simulink model "Neurofeedback_Fuzzy_MISO_Full_cute"  (R2022a)
settings: Solver=VariableStepAuto  StartTime=0.0  StopTime=90  RelTol=1e-3
libraries: simulink x5, dspsrcs4 x4, fuzblock x1
settings Model: Creator=mdls3  LastModifiedBy=mariodelossantos

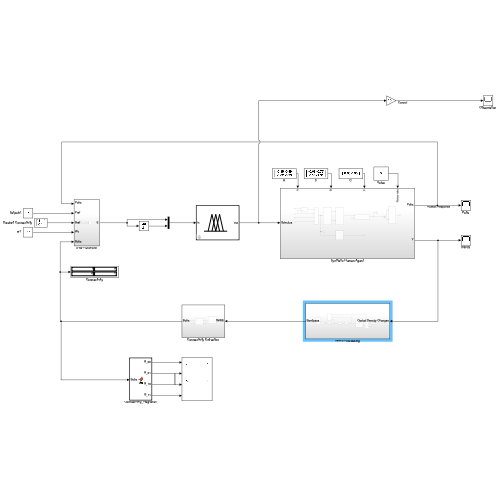
[thumbnail: Simulink's stored preview of the top-level diagram]
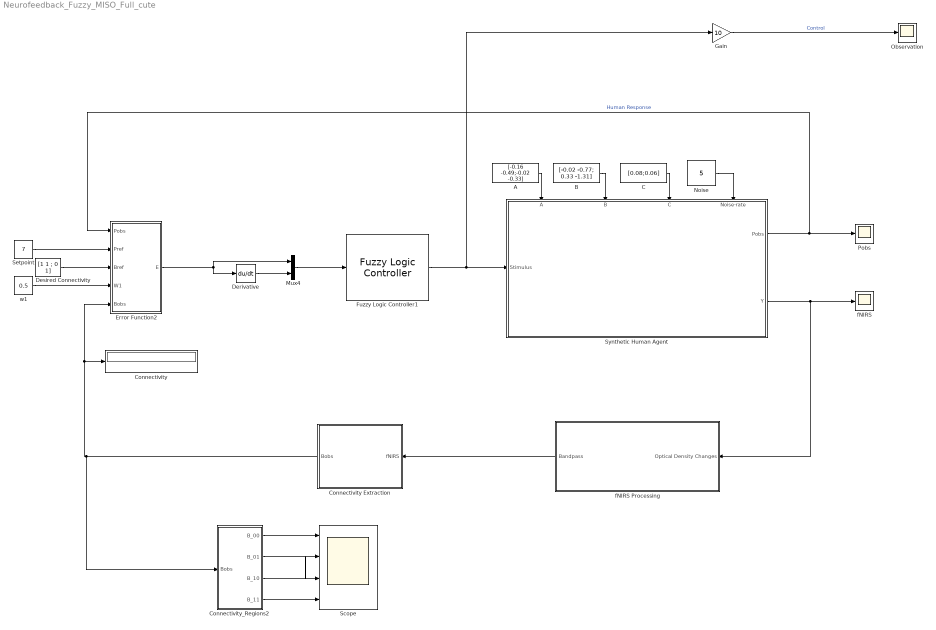
== system Neurofeedback_Fuzzy_MISO_Full_cute ==
  A : Constant  Value=[-0.16 -0.49;-0.02 -0.33]
  B : Constant  Value=[-0.02 -0.77; 0.33 -1.31]
  C : Constant  Value=[0.08;0.06]
  Connectivity : Display
  Connectivity Extraction : Subsystem
  Connectivity_Regions2 : MATLAB Function  TreatAsAtomicUnit=on
  Derivative : Derivative  CoefficientInTFapproximation=1
  Desired Connectivity : Constant  Value="[1   1 ; 0 1]"
  Error Function2 : Subsystem
  Fuzzy Logic Controller1 : fuzblock/Fuzzy Logic  Controller  FIS=cFNIRS_MISO_v3  OutputSampleNumber=101  DataType=double  FuzzifiedInputs=off  RuleFiringStrengths=off  RuleOutputs=off  AggregatedOutputs=off  SimulateUsing=Interpreted execution  OutOfRangeInputValueMessage=warning  NoRuleFiredMessage=warning  EmptyOutputFuzzySetMessage=warning
  Gain : Gain  Gain=10
  Mux4 : Mux  Inputs=2
  Noise : Constant  Value=5
  Observation : Scope
  Pobs : Scope
  Scope : Scope  NumInputPorts=4
  Setpoint : Constant  Value=7
  Synthetic Human Agent : Subsystem
      settings: PortSchema="{\"entries\":[{\"content\":{\"sides\":[{\"content\":{\"connectorIds\":[\"In1\"]},\"type\":\"ConnectorPlacement.EquallySpacedRectSide\",\"uuid\":\"bfbcc5e8-6241-430f-b542-d1842988c81e\"},{\"content\":{\"connectorIds\":[\"Out1\",\"Out2\"],\"side\":\"RIGHT\"},\"type\":\"ConnectorPlacement.EquallySpacedRectSide\",\"uuid\":\"5787ae13-1686-4c0f-bd71-92bd424cb6c3\"},{\"content\":{\"connectorIds\":[\"In2\",\"In3\",\"In4\",\"In5\"],\"side\":\"TOP\"},\"type\":\"ConnectorPlacement.EquallySpacedRectSide\",\"uuid\":\"d1dd531e-b262-408a-a912-471f5b03e825\"}]},\"type\":\"ConnectorPlacement.EquallySpacedConnector\",\"uuid\":\"b2c21004-90c2-4258-a219-9564d29dafe7\"}],\"packageUris\":[\"http://schema.mathworks.com/mf0/Connector/R2020b\"],\"version\":\"1.0\"}"
  fNIRS : Scope
  fNIRS Processing : Subsystem
  w1 : Constant  Value=0.5
  wires:
  Error Function2/1(E) -> Mux4/1, Derivative/1
  Synthetic Human Agent/2(Y) -> fNIRS/1, fNIRS Processing/1(Optical Density Changes)
  Noise/1 -> Synthetic Human Agent/5(Noise-rate)
  Derivative/1 -> Mux4/2
  Setpoint/1 -> Error Function2/2(Pref)
  Synthetic Human Agent/1(Pobs) -> Error Function2/1(Pobs), Pobs/1  "Human Response"
  Mux4/1 -> Fuzzy Logic Controller1/1
  A/1 -> Synthetic Human Agent/2(A)
  w1/1 -> Error Function2/4(W1)
  Desired Connectivity/1 -> Error Function2/3(Bref)
  C/1 -> Synthetic Human Agent/4(C)
  B/1 -> Synthetic Human Agent/3(B)
  Fuzzy Logic Controller1/1 -> Gain/1, Synthetic Human Agent/1(Stimulus)
  fNIRS Processing/1(Bandpass) -> Connectivity Extraction/1(fNIRS)
  Connectivity_Regions2/4(B_11) -> Scope/4
  Connectivity_Regions2/2(B_01) -> Scope/3
  Connectivity_Regions2/1(B_00) -> Scope/1
  Connectivity Extraction/1(Bobs) -> Connectivity_Regions2/1(Bobs), Error Function2/5(Bobs), Connectivity/1
  Connectivity_Regions2/3(B_10) -> Scope/2
  Gain/1 -> Observation/1  "Control"

== system Neurofeedback_Fuzzy_MISO_Full_cute/Connectivity Extraction ==
  fNIRS : Inport
  DQ1 : Scope
  Incremental_Avg_Boot1 : Subsystem
  Threshold : Constant  Value=0.6
  getConnectivity : MATLAB Function  TreatAsAtomicUnit=on  SystemSampleTime=0
  Bobs : Outport
  wires:
  getConnectivity/2(DQ) -> DQ1/1
  Incremental_Avg_Boot1/1("D ") -> getConnectivity/1("D ")
  Threshold/1 -> getConnectivity/2(Threshold)
  fNIRS/1 -> Incremental_Avg_Boot1/1(fNIRS)
  getConnectivity/1(Bobs) -> Bobs/1

== system Neurofeedback_Fuzzy_MISO_Full_cute/Error Function2 ==
  Pobs : Inport
  Pref : Inport  Port=2
  Bref : Inport  Port=3
  W1 : Inport  Port=4
  Bobs : Inport  Port=5
  Error Function : Subsystem
  Rehabilitation Train : Subsystem
  E : Outport
  wires:
  Bref/1 -> Error Function/3(Bref)
  Bobs/1 -> Error Function/4(Bobs)
  W1/1 -> Error Function/5(W1)
  Pref/1 -> Rehabilitation Train/1(In1)
  Pobs/1 -> Error Function/1(Pobs)
  Rehabilitation Train/1(Instruction) -> Error Function/2(Pref)
  Error Function/1(E) -> E/1

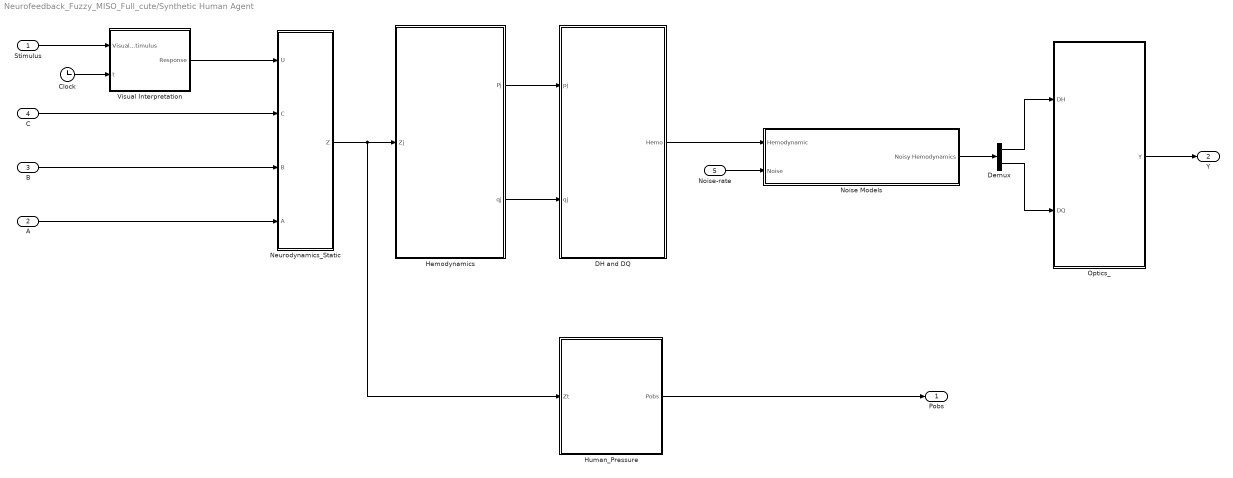
== system Neurofeedback_Fuzzy_MISO_Full_cute/Synthetic Human Agent ==
  Stimulus : Inport
  A : Inport  Port=2
  B : Inport  Port=3
  C : Inport  Port=4
  Noise-rate : Inport  Port=5
  Clock : Clock
  DH and DQ : Subsystem
  Demux : Demux  Outputs=2
  Hemodynamics : Subsystem
  Human_Pressure : Subsystem
  Neurodynamics_Static : Subsystem
  Noise Models : Subsystem
  Optics_ : MATLAB Function  TreatAsAtomicUnit=on
  Visual Interpretation : MATLAB Function  TreatAsAtomicUnit=on
  Pobs : Outport
  Y : Outport  Port=2
  wires:
  DH and DQ/1(Hemo) -> Noise Models/1(Hemodynamic)
  Hemodynamics/1(Pj) -> DH and DQ/1(pj)
  C/1 -> Neurodynamics_Static/2(C)
  Hemodynamics/2(qj) -> DH and DQ/2(qj)
  A/1 -> Neurodynamics_Static/4(A)
  Human_Pressure/1(Pobs) -> Pobs/1
  B/1 -> Neurodynamics_Static/3(B)
  Neurodynamics_Static/1(Z) -> Human_Pressure/1(Zt), Hemodynamics/1(Zj)
  Clock/1 -> Visual Interpretation/2(t)
  Stimulus/1 -> Visual Interpretation/1(Visual_Stimulus)
  Visual Interpretation/1(Response) -> Neurodynamics_Static/1(U)
  Noise Models/1(Noisy Hemodynamics) -> Demux/1
  Noise-rate/1 -> Noise Models/2(Noise)
  Demux/1 -> Optics_/1(DH)
  Demux/2 -> Optics_/2(DQ)
  Optics_/1(Y) -> Y/1

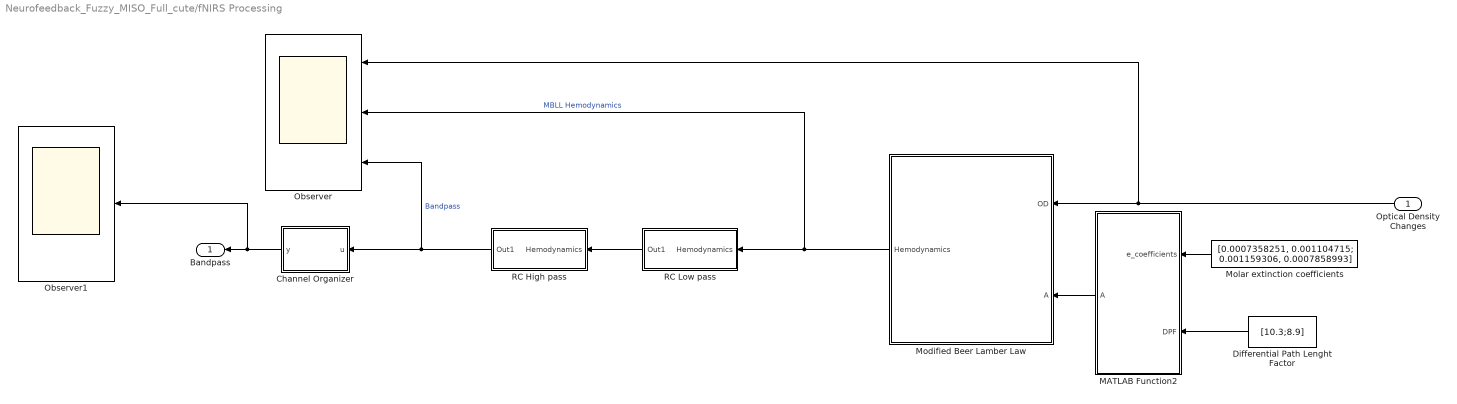
== system Neurofeedback_Fuzzy_MISO_Full_cute/fNIRS Processing ==
  Optical Density Changes : Inport
  Channel Organizer : MATLAB Function  TreatAsAtomicUnit=on
  Differential Path Lenght Factor : Constant  Value=[10.3;8.9]
  MATLAB Function2 : MATLAB Function  TreatAsAtomicUnit=on
  Modified Beer Lamber Law : MATLAB Function  TreatAsAtomicUnit=on
  Molar extinction coefficients : Constant  Value=|
      | [0.0007358251, 0.001104715;
      | 0.001159306, 0.0007858993]
  Observer : Scope  NumInputPorts=3
  Observer1 : Scope
  RC High pass : Subsystem
  RC Low pass : Subsystem
  Bandpass : Outport
  wires:
  Modified Beer Lamber Law/1(Hemodynamics) -> Observer/2, RC Low pass/1(Hemodynamics)  "MBLL Hemodynamics"
  Optical Density Changes/1 -> Modified Beer Lamber Law/1(OD), Observer/1
  RC High pass/1(Out1) -> Channel Organizer/1(u), Observer/3  "Bandpass"
  MATLAB Function2/1(A) -> Modified Beer Lamber Law/2(A)
  Differential Path Lenght Factor/1 -> MATLAB Function2/2(DPF)
  Molar extinction coefficients/1 -> MATLAB Function2/1(e_coefficients)
  Channel Organizer/1(y) -> Observer1/1, Bandpass/1
  RC Low pass/1(Out1) -> RC High pass/1(Hemodynamics)

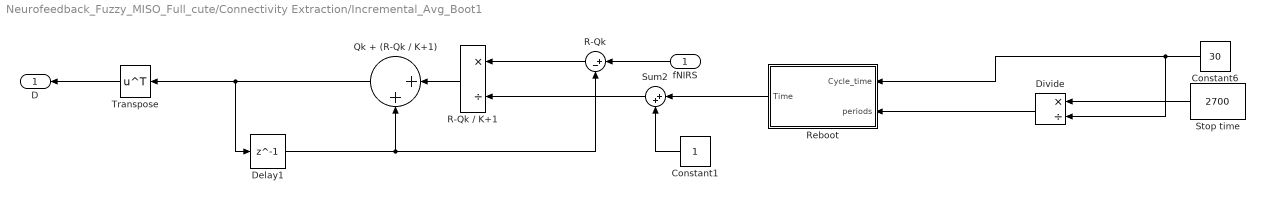
== system Neurofeedback_Fuzzy_MISO_Full_cute/Connectivity Extraction/Incremental_Avg_Boot1 ==
  fNIRS : Inport
  Constant1 : Constant
  Constant6 : Constant  Value=30
  Delay1 : Delay  DelayLength=1  InitialCondition=[0; 0; 0; 0]
  Divide : Product  Inputs=*/
  "Qk + (R-Qk / K+1) " : Sum  Inputs=|++
  R-Qk : Sum  Inputs=|+-
  R-Qk / K+1 : Product  Inputs=*/
  Reboot : Subsystem
  Stop time : Constant  Value=2700
  Sum2 : Sum  Inputs=|++
  Transpose : Math  Operator=transpose
  "D " : Outport
  wires:
  Constant1/1 -> Sum2/2
  fNIRS/1 -> R-Qk/1
  R-Qk / K+1/1 -> "Qk + (R-Qk / K+1) "/1
  Sum2/1 -> R-Qk / K+1/2
  R-Qk/1 -> R-Qk / K+1/1
  Delay1/1 -> R-Qk/2, "Qk + (R-Qk / K+1) "/2
  Reboot/1(Time) -> Sum2/1
  Constant6/1 -> Divide/2, Reboot/1(Cycle_time)
  Divide/1 -> Reboot/2(periods)
  Stop time/1 -> Divide/1
  "Qk + (R-Qk / K+1) "/1 -> Transpose/1, Delay1/1
  Transpose/1 -> "D "/1

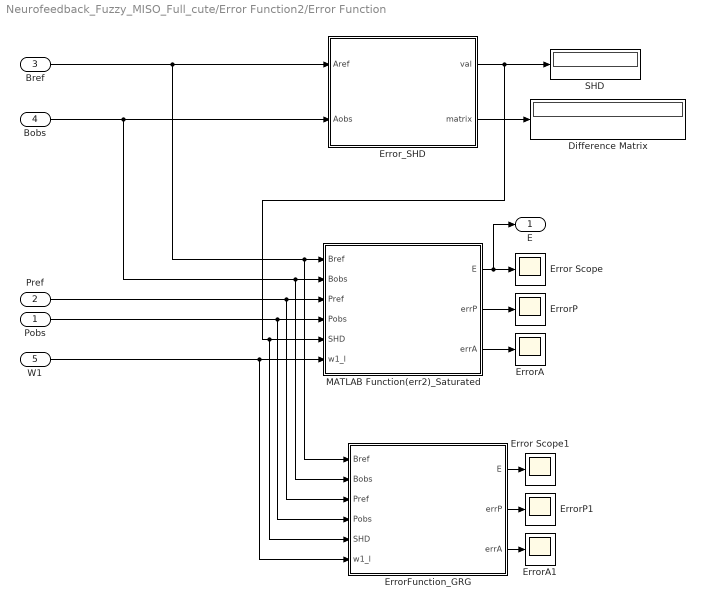
== system Neurofeedback_Fuzzy_MISO_Full_cute/Error Function2/Error Function ==
  Pobs : Inport
  Pref : Inport  Port=2
  Bref : Inport  Port=3
  Bobs : Inport  Port=4
  W1 : Inport  Port=5
  Difference Matrix : Display
  Error Scope : Scope
  Error Scope1 : Scope
  ErrorA : Scope
  ErrorA1 : Scope
  ErrorFunction_GRG : MATLAB Function  TreatAsAtomicUnit=on
  ErrorP : Scope
  ErrorP1 : Scope
  Error_SHD : MATLAB Function  TreatAsAtomicUnit=on
  MATLAB Function(err2)_Saturated : MATLAB Function  TreatAsAtomicUnit=on
  SHD : Display
  E : Outport
  wires:
  Error_SHD/2(matrix) -> Difference Matrix/1
  Bref/1 -> ErrorFunction_GRG/1(Bref), MATLAB Function(err2)_Saturated/1(Bref), Error_SHD/1(Aref)
  Error_SHD/1(val) -> ErrorFunction_GRG/5(SHD), MATLAB Function(err2)_Saturated/5(SHD), SHD/1
  Bobs/1 -> ErrorFunction_GRG/2(Bobs), MATLAB Function(err2)_Saturated/2(Bobs), Error_SHD/2(Aobs)
  Pref/1 -> ErrorFunction_GRG/3(Pref), MATLAB Function(err2)_Saturated/3(Pref)
  W1/1 -> MATLAB Function(err2)_Saturated/6(w1_l), ErrorFunction_GRG/6(w1_l)
  MATLAB Function(err2)_Saturated/1(E) -> E/1, Error Scope/1
  Pobs/1 -> ErrorFunction_GRG/4(Pobs), MATLAB Function(err2)_Saturated/4(Pobs)
  MATLAB Function(err2)_Saturated/2(errP) -> ErrorP/1
  MATLAB Function(err2)_Saturated/3(errA) -> ErrorA/1
  ErrorFunction_GRG/2(errP) -> ErrorP1/1
  ErrorFunction_GRG/3(errA) -> ErrorA1/1
  ErrorFunction_GRG/1(E) -> Error Scope1/1

== system Neurofeedback_Fuzzy_MISO_Full_cute/Error Function2/Rehabilitation Train ==
  In1 : Inport
  Duty_Cycle_U1 : Constant  Value=0.1666666666666667  OutMin=[0]  OutMax=[0.8]
  Period_Time_U1 : Constant  Value=30
  Setpoint_follow : Product
  Variable Pulse Generator2 : VariablePulseGenerator  AllowZeroPulseWidth=on  RunAtFixedTimeIntervals=on  SampleTime=1/10
  Instruction : Outport
  wires:
  Duty_Cycle_U1/1 -> Variable Pulse Generator2/1
  In1/1 -> Setpoint_follow/2
  Period_Time_U1/1 -> Variable Pulse Generator2/2
  Setpoint_follow/1 -> Instruction/1
  Variable Pulse Generator2/1 -> Setpoint_follow/1

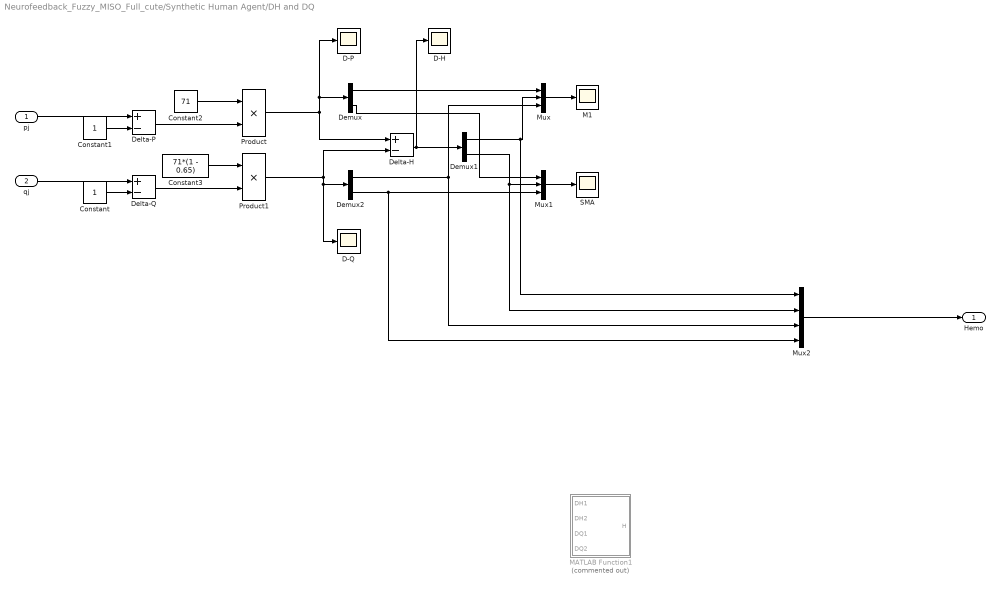
== system Neurofeedback_Fuzzy_MISO_Full_cute/Synthetic Human Agent/DH and DQ ==
  pj : Inport
  qj : Inport  Port=2
  Constant : Constant
  Constant1 : Constant
  Constant2 : Constant  Value=71
  Constant3 : Constant  Value=71*(1 - 0.65)
  D-H : Scope
  D-P : Scope
  D-Q : Scope
  Delta-H : Sum  Inputs=+-
  Delta-P : Sum  Inputs=+-
  Delta-Q : Sum  Inputs=+-
  Demux : Demux  Outputs=2
  Demux1 : Demux  Outputs=2
  Demux2 : Demux  Outputs=2
  M1 : Scope
  MATLAB Function1 : MATLAB Function  Commented=on  TreatAsAtomicUnit=on
  Mux : Mux  Inputs=3
  Mux1 : Mux  Inputs=3
  Mux2 : Mux
  Product : Product
  Product1 : Product
  SMA : Scope
  Hemo : Outport
  wires:
  Constant2/1 -> Product/1
  Delta-Q/1 -> Product1/2
  Constant3/1 -> Product1/1
  Demux2/2 -> Mux2/4, Mux1/3
  pj/1 -> Delta-P/1
  Mux1/1 -> SMA/1
  Demux/2 -> Mux1/1
  Mux/1 -> M1/1
  Constant/1 -> Delta-Q/2
  Delta-P/1 -> Product/2
  Product1/1 -> Demux2/1, D-Q/1, Delta-H/2
  qj/1 -> Delta-Q/1
  Demux/1 -> Mux/1
  Delta-H/1 -> Demux1/1, D-H/1
  Demux1/1 -> Mux2/1, Mux/2
  Demux1/2 -> Mux2/2, Mux1/2
  Product/1 -> Demux/1, D-P/1, Delta-H/1
  Demux2/1 -> Mux2/3, Mux/3
  Constant1/1 -> Delta-P/2
  Mux2/1 -> Hemo/1

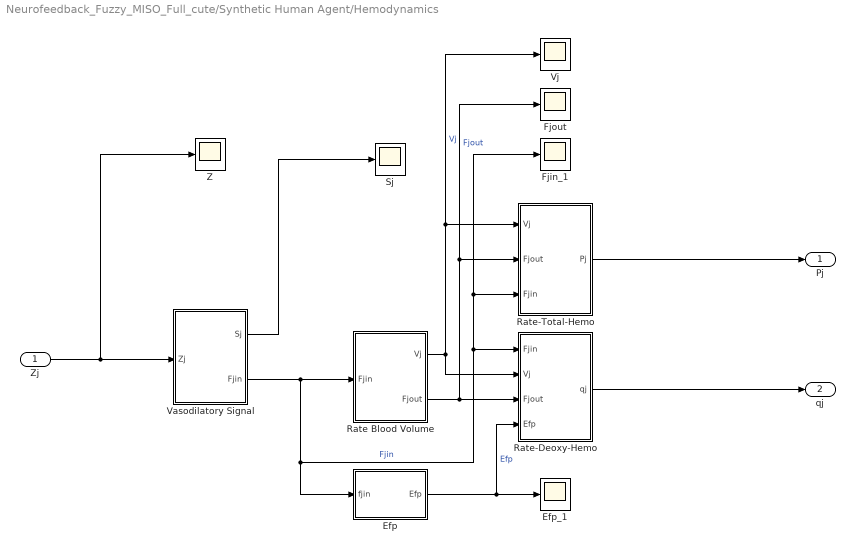
== system Neurofeedback_Fuzzy_MISO_Full_cute/Synthetic Human Agent/Hemodynamics ==
  Zj : Inport
  Efp : MATLAB Function  TreatAsAtomicUnit=on
  Efp_1 : Scope
  Fjin_1 : Scope
  Fjout : Scope
  Rate Blood Volume : Subsystem
  Rate-Deoxy-Hemo : Subsystem
  Rate-Total-Hemo : Subsystem
  Sj : Scope
  Vasodilatory Signal : Subsystem
  Vj : Scope
  Z : Scope
  Pj : Outport
  qj : Outport  Port=2
  wires:
  Rate-Deoxy-Hemo/1(qj) -> qj/1
  Zj/1 -> Vasodilatory Signal/1(Zj), Z/1
  Vasodilatory Signal/1(Sj) -> Sj/1
  Rate Blood Volume/2(Fjout) -> Fjout/1, Rate-Total-Hemo/2(Fjout), Rate-Deoxy-Hemo/3(Fjout)  "Fjout"
  Rate Blood Volume/1(Vj) -> Vj/1, Rate-Total-Hemo/1(Vj), Rate-Deoxy-Hemo/2(Vj)  "Vj"
  Rate-Total-Hemo/1(Pj) -> Pj/1
  Efp/1(Efp) -> Rate-Deoxy-Hemo/4(Efp), Efp_1/1  "Efp"
  Vasodilatory Signal/2(Fjin) -> Efp/1(fjin), Fjin_1/1, Rate-Total-Hemo/3(Fjin), Rate-Deoxy-Hemo/1(Fjin), Rate Blood Volume/1(Fjin)  "Fjin"

== system Neurofeedback_Fuzzy_MISO_Full_cute/Synthetic Human Agent/Human_Pressure ==
  Zt : Inport
  Clock : Clock
  Gain : Gain  Gain=10
  Pressure Generator : MATLAB Function  TreatAsAtomicUnit=on
  SENSOR : MATLAB Function  TreatAsAtomicUnit=on
  Scope : Scope
  Scope1 : Scope
  Pobs : Outport
  wires:
  Clock/1 -> Pressure Generator/2(t)
  Zt/1 -> Pressure Generator/1(Zt)
  SENSOR/1(Pobs) -> Scope1/1, Gain/1
  Pressure Generator/1(Pobs) -> SENSOR/1(Vout), Scope/1
  Gain/1 -> Pobs/1

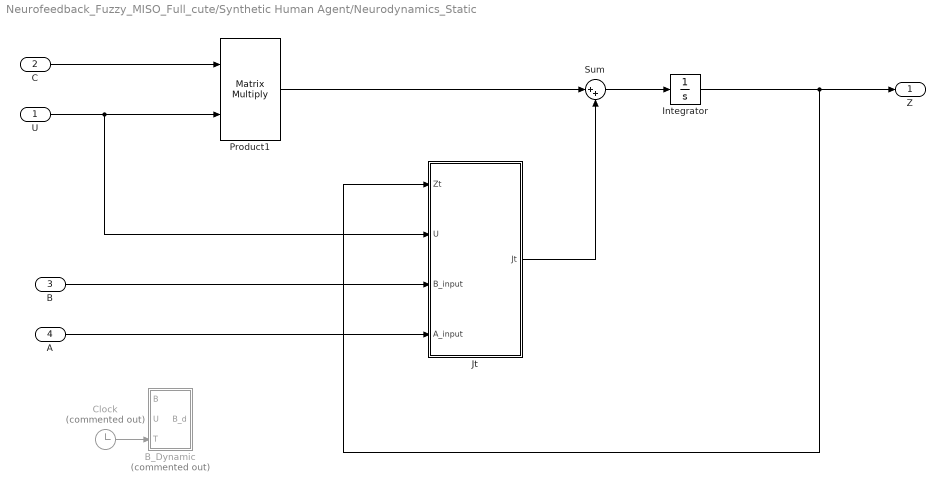
== system Neurofeedback_Fuzzy_MISO_Full_cute/Synthetic Human Agent/Neurodynamics_Static ==
  U : Inport
  C : Inport  Port=2
  B : Inport  Port=3
  A : Inport  Port=4
  B_Dynamic : Subsystem  Commented=on
  Clock : Clock  Commented=on
  Integrator : Integrator
  Jt : MATLAB Function  TreatAsAtomicUnit=on
  Product1 : Product  Multiplication=Matrix(*)
  Sum : Sum  Inputs=|++
  Z : Outport
  wires:
  Integrator/1 -> Jt/1(Zt), Z/1
  Product1/1 -> Sum/1
  Jt/1(Jt) -> Sum/2
  Sum/1 -> Integrator/1
  U/1 -> Product1/2, Jt/2(U)
  C/1 -> Product1/1
  A/1 -> Jt/4(A_input)
  Clock/1 -> B_Dynamic/3(T)
  B/1 -> Jt/3(B_input)

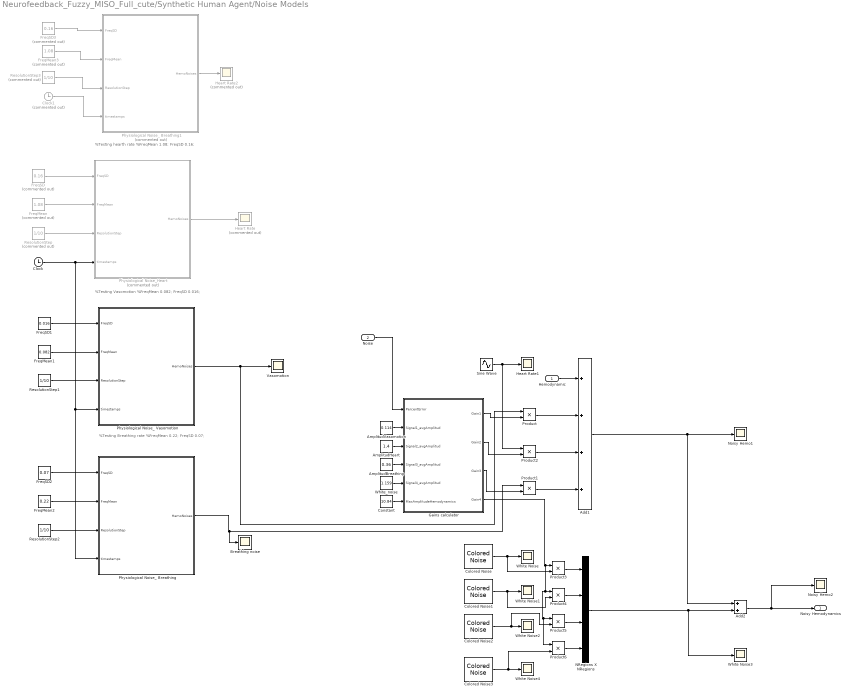
== system Neurofeedback_Fuzzy_MISO_Full_cute/Synthetic Human Agent/Noise Models ==
  note: %Testing hearth rate
      | %FreqMean 1.08; FreqSD 0.16;
  note: %Testing Breathing rate
      | %FreqMean 0.22; FreqSD 0.07;
  note: %Testing Vasomotion
      | %FreqMean 0.082; FreqSD 0.016;
  Hemodynamic : Inport
  Noise : Inport  Port=2
  Add1 : Sum  Inputs=++++
  Add2 : Sum
  AmplitudBreathing : Constant  Value=0.36
  AmplitudHeart : Constant  Value=1.4
  AmplitudVasomotion : Constant  Value=0.114
  Breathing noise : Scope
  Clock : Clock
  Clock1 : Clock  Commented=on
  Colored Noise : dspsrcs4/Colored Noise  Color=white  InverseFrequencyPower=1  BoundedOutput=on  NumChannels=1  OutputDataType=double  SamplesPerFrame=1  SampleTime=1/10  RandomStream=mt19937ar with seed  Seed=67  SimulateUsing=Interpreted execution
      settings: SourceProductBaseCode=DS
  Colored Noise1 : dspsrcs4/Colored Noise  Color=white  InverseFrequencyPower=1  BoundedOutput=on  NumChannels=1  OutputDataType=double  SamplesPerFrame=1  SampleTime=1/10  RandomStream=mt19937ar with seed  Seed=40  SimulateUsing=Interpreted execution
      settings: SourceProductBaseCode=DS
  Colored Noise2 : dspsrcs4/Colored Noise  Color=white  InverseFrequencyPower=1  BoundedOutput=on  NumChannels=1  OutputDataType=double  SamplesPerFrame=1  SampleTime=1/10  RandomStream=mt19937ar with seed  Seed=41  SimulateUsing=Interpreted execution
      settings: SourceProductBaseCode=DS
  Colored Noise3 : dspsrcs4/Colored Noise  Color=white  InverseFrequencyPower=1  BoundedOutput=on  NumChannels=1  OutputDataType=double  SamplesPerFrame=1  SampleTime=1/10  RandomStream=mt19937ar with seed  Seed=50  SimulateUsing=Interpreted execution
      settings: SourceProductBaseCode=DS
  Constant : Constant  Value=10.84
  FreqMean : Constant  Commented=on  Value=1.08
  FreqMean1 : Constant  Value=0.082
  FreqMean2 : Constant  Value=0.22
  FreqMean3 : Constant  Commented=on  Value=1.08
  FreqSD : Constant  Commented=on  Value=0.16
  FreqSD1 : Constant  Value=0.016
  FreqSD2 : Constant  Value=0.07
  FreqSD3 : Constant  Commented=on  Value=0.16
  Gains calculator : MATLAB Function  TreatAsAtomicUnit=on
  Heart Rate : Scope  Commented=on
  Heart Rate1 : Scope
  Heart Rate2 : Scope  Commented=on
  NRegions X NRegions : Mux
  Noisy Hemo1 : Scope
  Noisy Hemo2 : Scope
  Physiological Noise_ Breathing : MATLAB Function  TreatAsAtomicUnit=on
  Physiological Noise_ Breathing1 : MATLAB Function  Commented=on  TreatAsAtomicUnit=on
  Physiological Noise_ Vasomotion : MATLAB Function  TreatAsAtomicUnit=on
  Physiological Noise_Heart : MATLAB Function  Commented=on  TreatAsAtomicUnit=on
  Product{,1..6} (7 alike) : Product
  ResolutionStep : Constant  Commented=on  Value=1/10
  ResolutionStep1 : Constant  Value=1/10
  ResolutionStep2 : Constant  Value=1/10
  ResolutionStep3 : Constant  Commented=on  Value=1/10
  Sine Wave : Sin  Frequency=1.08 * 2*pi  SampleTime=0
  Vasomotion : Scope
  White Noise{,1..4} (5 alike) : Scope
  White_noise : Constant  Value=1.159
  Noisy Hemodynamics : Outport
  wires:
  FreqSD/1 -> Physiological Noise_Heart/1(FreqSD)
  FreqMean/1 -> Physiological Noise_Heart/2(FreqMean)
  ResolutionStep/1 -> Physiological Noise_Heart/3(ResolutionStep)
  ResolutionStep1/1 -> Physiological Noise_ Vasomotion/3(ResolutionStep)
  FreqSD1/1 -> Physiological Noise_ Vasomotion/1(FreqSD)
  Clock/1 -> Physiological Noise_Heart/4(timestamps), Physiological Noise_ Breathing/4(timestamps), Physiological Noise_ Vasomotion/4(timestamps)
  FreqMean1/1 -> Physiological Noise_ Vasomotion/2(FreqMean)
  Physiological Noise_ Breathing/1(HemoNoises) -> Product1/1, Breathing noise/1
  ResolutionStep2/1 -> Physiological Noise_ Breathing/3(ResolutionStep)
  FreqMean2/1 -> Physiological Noise_ Breathing/2(FreqMean)
  FreqSD2/1 -> Physiological Noise_ Breathing/1(FreqSD)
  Physiological Noise_ Vasomotion/1(HemoNoises) -> Product/1, Vasomotion/1
  Physiological Noise_Heart/1(HemoNoises) -> Heart Rate/1
  Physiological Noise_ Breathing1/1(HemoNoises) -> Heart Rate2/1
  Clock1/1 -> Physiological Noise_ Breathing1/4(timestamps)
  FreqSD3/1 -> Physiological Noise_ Breathing1/1(FreqSD)
  FreqMean3/1 -> Physiological Noise_ Breathing1/2(FreqMean)
  ResolutionStep3/1 -> Physiological Noise_ Breathing1/3(ResolutionStep)
  Sine Wave/1 -> Product2/1, Heart Rate1/1
  Gains calculator/1(Gain1) -> Product/2
  Add1/1 -> Add2/1, Noisy Hemo1/1
  AmplitudVasomotion/1 -> Gains calculator/2(Signal1_avgAmplitud)
  Hemodynamic/1 -> Add1/1
  Constant/1 -> Gains calculator/6(MaxAmplitudeHemodynamics)
  Gains calculator/2(Gain2) -> Product2/2
  Gains calculator/3(Gain3) -> Product1/2
  AmplitudHeart/1 -> Gains calculator/3(Signal2_avgAmplitud)
  AmplitudBreathing/1 -> Gains calculator/4(Signal3_avgAmplitud)
  Colored Noise/1 -> Product3/2, White Noise/1
  Colored Noise1/1 -> Product4/2, White Noise1/1
  Colored Noise2/1 -> Product5/2, White Noise2/1
  NRegions X NRegions/1 -> White Noise3/1, Add2/2
  Colored Noise3/1 -> Product6/2, White Noise4/1
  Add2/1 -> Noisy Hemodynamics/1, Noisy Hemo2/1
  Product/1 -> Add1/2
  Product2/1 -> Add1/3
  Product1/1 -> Add1/4
  Product3/1 -> NRegions X NRegions/1
  White_noise/1 -> Gains calculator/5(Signal4_avgAmplitud)
  Gains calculator/4(Gain4) -> Product6/1, Product5/1, Product4/1, Product3/1
  Product4/1 -> NRegions X NRegions/2
  Product5/1 -> NRegions X NRegions/3
  Product6/1 -> NRegions X NRegions/4
  Noise/1 -> Gains calculator/1(PercentError)

== system Neurofeedback_Fuzzy_MISO_Full_cute/fNIRS Processing/RC High pass ==
  Hemodynamics : Inport
  Add : Sum  Inputs=+-
  Discrete Derivative : simulink/Discrete/Discrete Derivative  gainval=0.1  ICPrevScaledInput=0.0  OutMin=[]  OutMax=[]  OutDataType=fixdt(1, 16)  OutScaling=2^-10  DoSatur=off
  Discrete Derivative1 : simulink/Discrete/Discrete Derivative  gainval=0.12  ICPrevScaledInput=0.0  OutMin=[]  OutMax=[]  OutDataType=fixdt(1, 16)  OutScaling=2^-10  DoSatur=off
  Gain : Gain  Gain=810
  RC High pass1 : Subsystem  Commented=on
  Out1 : Outport
  wires:
  Add/1 -> Gain/1
  Gain/1 -> Discrete Derivative/1, Out1/1
  Discrete Derivative/1 -> Add/2
  Discrete Derivative1/1 -> Add/1
  Hemodynamics/1 -> Discrete Derivative1/1  "Bandpass"

== system Neurofeedback_Fuzzy_MISO_Full_cute/fNIRS Processing/RC Low pass ==
  Hemodynamics : Inport
  Add : Sum  Inputs=+-
  Discrete Derivative : simulink/Discrete/Discrete Derivative  gainval=3.2  ICPrevScaledInput=0.0  OutMin=[]  OutMax=[]  OutDataType=fixdt(1, 16)  OutScaling=2^-10  DoSatur=off
  Out1 : Outport
  wires:
  Hemodynamics/1 -> Add/1
  Discrete Derivative/1 -> Add/2
  Add/1 -> Discrete Derivative/1, Out1/1

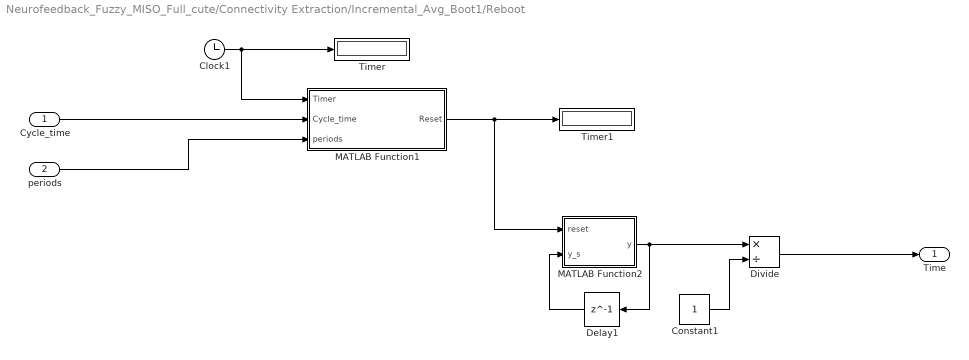
== system Neurofeedback_Fuzzy_MISO_Full_cute/Connectivity Extraction/Incremental_Avg_Boot1/Reboot ==
  Cycle_time : Inport
  periods : Inport  Port=2
  Clock1 : Clock
  Constant1 : Constant
  Delay1 : Delay  DelayLength=1
  Divide : Product  Inputs=*/
  MATLAB Function1 : MATLAB Function  TreatAsAtomicUnit=on
  MATLAB Function2 : MATLAB Function  TreatAsAtomicUnit=on
  Timer : Display
  Timer1 : Display
  Time : Outport
  wires:
  MATLAB Function1/1(Reset) -> MATLAB Function2/1(reset), Timer1/1
  MATLAB Function2/1(y) -> Divide/1, Delay1/1
  Constant1/1 -> Divide/2
  Clock1/1 -> MATLAB Function1/1(Timer), Timer/1
  periods/1 -> MATLAB Function1/3(periods)
  Delay1/1 -> MATLAB Function2/2(y_s)
  Divide/1 -> Time/1
  Cycle_time/1 -> MATLAB Function1/2(Cycle_time)

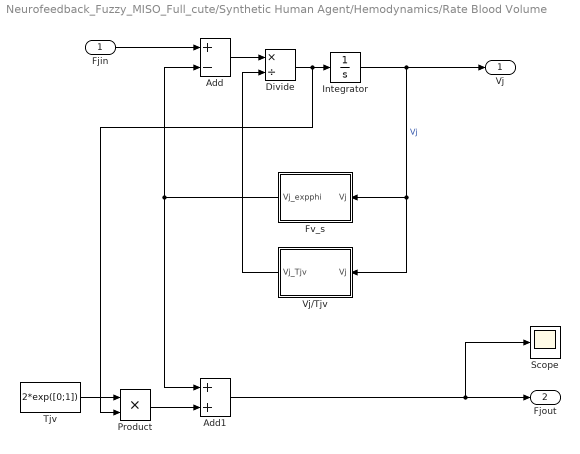
== system Neurofeedback_Fuzzy_MISO_Full_cute/Synthetic Human Agent/Hemodynamics/Rate Blood Volume ==
  Fjin : Inport
  Add : Sum  Inputs=+-
  Add1 : Sum
  Divide : Product  Inputs=*/
  Fv_s : MATLAB Function  TreatAsAtomicUnit=on
  Integrator : Integrator  InitialCondition=exp([0;0])
  Product : Product
  Scope : Scope
  Tjv : Constant  Value=2*exp([0;1])
  Vj/Tjv : MATLAB Function  TreatAsAtomicUnit=on
  Vj : Outport
  Fjout : Outport  Port=2
  wires:
  Fjin/1 -> Add/1
  Integrator/1 -> Vj/1, Vj/Tjv/1(Vj), Fv_s/1(Vj)  "Vj"
  Divide/1 -> Product/2, Integrator/1
  Fv_s/1(Vj_expphi) -> Add/2, Add1/1
  Add/1 -> Divide/1
  Vj/Tjv/1(Vj_Tjv) -> Divide/2
  Product/1 -> Add1/2
  Tjv/1 -> Product/1
  Add1/1 -> Scope/1, Fjout/1

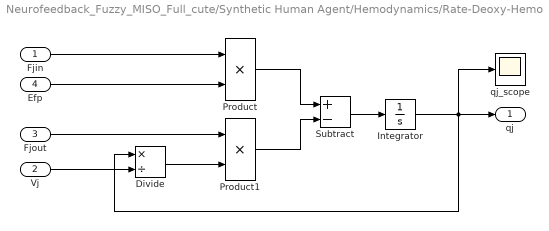
== system Neurofeedback_Fuzzy_MISO_Full_cute/Synthetic Human Agent/Hemodynamics/Rate-Deoxy-Hemo ==
  Fjin : Inport
  Vj : Inport  Port=2
  Fjout : Inport  Port=3
  Efp : Inport  Port=4
  Divide : Product  Inputs=*/
  Integrator : Integrator  InitialCondition=exp([0;0])
  Product : Product
  Product1 : Product
  Subtract : Sum  Inputs=+-
  qj_scope : Scope
  qj : Outport
  wires:
  Efp/1 -> Product/2
  Divide/1 -> Product1/2
  Subtract/1 -> Integrator/1
  Integrator/1 -> qj/1, Divide/1, qj_scope/1
  Vj/1 -> Divide/2
  Product1/1 -> Subtract/2
  Fjin/1 -> Product/1
  Fjout/1 -> Product1/1
  Product/1 -> Subtract/1

== system Neurofeedback_Fuzzy_MISO_Full_cute/Synthetic Human Agent/Hemodynamics/Rate-Total-Hemo ==
  Vj : Inport
  Fjout : Inport  Port=2
  Fjin : Inport  Port=3
  Divide : Product  Inputs=*/
  Integrator : Integrator  InitialCondition=exp([0;0])
  Product : Product
  Subtract : Sum  Inputs=+-
  pj : Scope
  Pj : Outport
  wires:
  Fjout/1 -> Subtract/2
  Product/1 -> Integrator/1
  Vj/1 -> Divide/2
  Subtract/1 -> Product/1
  Fjin/1 -> Subtract/1
  Divide/1 -> Product/2
  Integrator/1 -> Pj/1, pj/1, Divide/1

== system Neurofeedback_Fuzzy_MISO_Full_cute/Synthetic Human Agent/Hemodynamics/Vasodilatory Signal ==
  Zj : Inport
  Add : Sum  Inputs=+--
  Add1 : Sum  Inputs=+-
  Constant1 : Constant
  Integrator : Integrator
  Integrator1 : Integrator  InitialCondition=exp([0;0])
  K : Gain  Gain=0.64*exp([0;0.05])
  Scope1 : Scope
  Yj : Gain  Gain=0.32*exp([0;0.05])
  Sj : Outport
  Fjin : Outport  Port=2
  wires:
  Add1/1 -> Yj/1
  K/1 -> Add/2  "Kj*Sj"
  Constant1/1 -> Add1/2
  Zj/1 -> Add/1
  Integrator1/1 -> Fjin/1, Scope1/1, Add1/1
  Integrator/1 -> Sj/1, K/1, Integrator1/1
  Add/1 -> Integrator/1
  Yj/1 -> Add/3  "Yj(Fjin - 1)"

== system Neurofeedback_Fuzzy_MISO_Full_cute/Synthetic Human Agent/Neurodynamics_Static/B_Dynamic ==
  B : Inport
  U : Inport  Port=2
  T : Inport  Port=3
  Delay : Delay  DelayLength=1  InitialCondition=0
  Delay1 : Delay  DelayLength=1  InitialCondition=0
  Display : Display
  Display1 : Display
  Display2 : Display
  MATLAB Function : MATLAB Function  TreatAsAtomicUnit=on
  B_d : Outport
  wires:
  MATLAB Function/2(Th) -> Delay/1, Display1/1
  B/1 -> MATLAB Function/1(B)
  MATLAB Function/1(B_d) -> Delay1/1, B_d/1, Display/1
  Delay/1 -> MATLAB Function/5(Th_O)
  T/1 -> MATLAB Function/3(T)
  U/1 -> MATLAB Function/2(U), Display2/1
  Delay1/1 -> MATLAB Function/4(B_D)

== system Neurofeedback_Fuzzy_MISO_Full_cute/fNIRS Processing/RC High pass/RC High pass1 ==
  Hemodynamics : Inport
  Add : Sum  Inputs=+-
  Discrete Derivative : simulink/Discrete/Discrete Derivative  gainval=1.2  ICPrevScaledInput=0.0  OutMin=[]  OutMax=[]  OutDataType=fixdt(1, 16)  OutScaling=2^-10  DoSatur=off
  Discrete Derivative1 : simulink/Discrete/Discrete Derivative  gainval=1.4  ICPrevScaledInput=0.0  OutMin=[]  OutMax=[]  OutDataType=fixdt(1, 16)  OutScaling=2^-10  DoSatur=off
  Gain : Gain  Gain=800
  Out1 : Outport
  wires:
  Add/1 -> Gain/1
  Gain/1 -> Discrete Derivative/1, Out1/1
  Discrete Derivative/1 -> Add/2
  Discrete Derivative1/1 -> Add/1
  Hemodynamics/1 -> Discrete Derivative1/1

== matlab function Neurofeedback_Fuzzy_MISO_Full_cute/Synthetic Human Agent/Noise Models/Gains calculator ==
  settings: updateMethod=DISCRETE
  data: PercentError input; Signal1_avgAmplitud input; Signal2_avgAmplitud input; Signal3_avgAmplitud input; Signal4_avgAmplitud input; Gain1 output; MaxAmplitudeHemodynamics input; Gain2 output; Gain3 output; Gain4 output
function [Gain1, Gain2, Gain3, Gain4]    = Noise_gains(PercentError, Signal1_avgAmplitud,Signal2_avgAmplitud ,Signal3_avgAmplitud,Signal4_avgAmplitud,MaxAmplitudeHemodynamics)

Gain1 = ((MaxAmplitudeHemodynamics / 100) * PercentError)/ Signal1_avgAmplitud;

Gain2 = ((MaxAmplitudeHemodynamics / 100) * PercentError)/ Signal2_avgAmplitud;

Gain3 = ((MaxAmplitudeHemodynamics / 100) * PercentError)/ Signal3_avgAmplitud;

Gain4 = ((MaxAmplitudeHemodynamics / 100) * PercentError)/ Signal4_avgAmplitud;

== matlab function Neurofeedback_Fuzzy_MISO_Full_cute/Synthetic Human Agent/Noise Models/Physiological Noise_ Breathing ==
  settings: updateMethod=DISCRETE
  data: FreqSD input; HemoNoises output; FreqMean input; ResolutionStep input; timestamps input
function HemoNoises  = Neurofeedback_PhysiologicalNoise(FreqSD, FreqMean, ResolutionStep, timestamps)
%% Version V1
% Authors - Mario De Los Santos, Felipe Orihuela-Espina, Javier
% Herrera-Vega, Javier Andreu-Pérez
% Date - July 18th, 2022
% Email - madlsh3517@gmail.com
% Based on: Elwell et. al., 1999. Oscillations in cerebal haemodynamics.
%
%% Input Parameters
% FreqSD - Frequency standard deviation of the physiological noise. Scalar
% FreqMean - Frequency Mean of the physiological noise. Scalar
% Resolution Step - Sampling rate. Scalar
% Timestamps - Time sequence for the stimulus train. <1 x simulationLength>
% NRegions - Number of regions activated. Scalar.
%% Output Parameters
% 
% HemoNoises -  Noise generation for the hemodynamics signals.
%               <NRegions x simulationLength>
%
%% 

%Variables to ADD the noises to the models. 
% These variables divide the hemodynamics 
% inputs depending on the number of regions.
HemoNoises = 0;

%Calculation of the operative ranges to use
Initial =  FreqMean - 2 * FreqSD;
Ending = FreqMean + 2 * FreqSD;
Calsize =  (Ending - Initial - ResolutionStep)/ResolutionStep;
FrequencySet = linspace(Initial, Ending, Calsize);

amplitudeScaling = 1;
for i = 1:Calsize
    s = rng; %Rebot random seeed 
    %Random Amplitude
    %Centralized gaussian in the dispersion mean 
    %A = 0;
    L = normrnd(FreqMean, FreqSD);
    A = amplitudeScaling * L;
  
    %Random phase
    theta = (2 * pi * L - pi );
  
    %Fundamental signal
    tmpSin = A * sin(pi * FrequencySet(1,i) * timestamps + theta);
    HemoNoises = HemoNoises + tmpSin;
end
%This section should be generalized but do the work for now.

== matlab function Neurofeedback_Fuzzy_MISO_Full_cute/Synthetic Human Agent/Visual Interpretation ==
  data: Visual_Stimulus input; Response output; t input
function Response = fcn(Visual_Stimulus, t)
    R=17.5; %Resistor [Ohms] 10k 
    C= 0.65; %Capacitor [Faradays] 1mF
    V= Visual_Stimulus; %Voltage or system reference;
    Vc = V * (1- exp(-t/(R*C))); % Voltage at the capacitor  
    
Response = Vc;

== matlab function Neurofeedback_Fuzzy_MISO_Full_cute/Synthetic Human Agent/Noise Models/Physiological Noise_ Breathing1 ==
  settings: updateMethod=DISCRETE
  data: FreqSD input; HemoNoises output; FreqMean input; ResolutionStep input; timestamps input
function HemoNoises  = Neurofeedback_PhysiologicalNoise(FreqSD, FreqMean, ResolutionStep, timestamps)
%% Version V1
% Authors - Mario De Los Santos, Felipe Orihuela-Espina, Javier
% Herrera-Vega, Javier Andreu-Pérez
% Date - July 18th, 2022
% Email - madlsh3517@gmail.com
% Based on: Elwell et. al., 1999. Oscillations in cerebal haemodynamics.
%
%% Input Parameters
% FreqSD - Frequency standard deviation of the physiological noise. Scalar
% FreqMean - Frequency Mean of the physiological noise. Scalar
% Resolution Step - Sampling rate. Scalar
% Timestamps - Time sequence for the stimulus train. <1 x simulationLength>
% NRegions - Number of regions activated. Scalar.
%% Output Parameters
% 
% HemoNoises -  Noise generation for the hemodynamics signals.
%               <NRegions x simulationLength>
%
%% 

%Variables to ADD the noises to the models. 
% These variables divide the hemodynamics 
% inputs depending on the number of regions.
HemoNoises = 0;

%Calculation of the operative ranges to use
Initial =  FreqMean - 2 * FreqSD;
Ending = FreqMean + 2 * FreqSD;
Calsize =  (Ending - Initial)/ResolutionStep;
FrequencySet = linspace(Initial, Ending, Calsize);

amplitudeScaling = 1;
for i = 1:Calsize
    s = rng; %Rebot random seeed 
    %Random Amplitude
    %Centralized gaussian in the dispersion mean 
    %A = 0;
    L = normrnd(FreqMean, FreqSD);
    A = amplitudeScaling * L;
  
    %Random phase
    theta = 0;
  
    %Fundamental signal
    tmpSin = A * sin((pi * FrequencySet(1,i) * timestamps + theta)*2*pi);
    HemoNoises = HemoNoises + tmpSin;
end
%This section should be generalized but do the work for now.

== matlab function Neurofeedback_Fuzzy_MISO_Full_cute/Synthetic Human Agent/Noise Models/Physiological Noise_ Vasomotion ==
  settings: updateMethod=DISCRETE
  data: FreqSD input; HemoNoises output; FreqMean input; ResolutionStep input; timestamps input
function HemoNoises  = Neurofeedback_PhysiologicalNoise(FreqSD, FreqMean, ResolutionStep, timestamps)
%% Version V1
% Authors - Mario De Los Santos, Felipe Orihuela-Espina, Javier
% Herrera-Vega, Javier Andreu-Pérez
% Date - July 18th, 2022
% Email - madlsh3517@gmail.com
% Based on: Elwell et. al., 1999. Oscillations in cerebal haemodynamics.
%
%% Input Parameters
% FreqSD - Frequency standard deviation of the physiological noise. Scalar
% FreqMean - Frequency Mean of the physiological noise. Scalar
% Resolution Step - Sampling rate. Scalar
% Timestamps - Time sequence for the stimulus train. <1 x simulationLength>
% NRegions - Number of regions activated. Scalar.
%% Output Parameters
% 
% HemoNoises -  Noise generation for the hemodynamics signals.
%               <NRegions x simulationLength>
%
%% 

%Variables to ADD the noises to the models. 
% These variables divide the hemodynamics 
% inputs depending on the number of regions.
HemoNoises = 0;

%Calculation of the operative ranges to use
Initial =  FreqMean - 2 * FreqSD;
Ending = FreqMean + 2 * FreqSD + ResolutionStep;
Calsize =  (Ending - Initial)/ResolutionStep;
FrequencySet = linspace(Initial, Ending, Calsize);

amplitudeScaling = 1;
for i = 1:Calsize
    s = rng; %Rebot random seeed 
    %Random Amplitude
    %Centralized gaussian in the dispersion mean 
    %A = 0;
    A = amplitudeScaling * normrnd(FreqMean,FreqSD);
    %A = amplitudeScaling * randn(1);
  
    %Random phase
    theta = (2 * pi * normrnd(FreqMean, FreqSD) - pi );
  
    %Fundamental signal
    tmpSin = A * sin(pi * FrequencySet(1,i) * timestamps + theta);
    HemoNoises = HemoNoises + tmpSin;
end
%This section should be generalized but do the work for now.

== matlab function Neurofeedback_Fuzzy_MISO_Full_cute/Synthetic Human Agent/Noise Models/Physiological Noise_Heart ==
  settings: updateMethod=DISCRETE
  data: FreqSD input; HemoNoises output; FreqMean input; ResolutionStep input; timestamps input
function HemoNoises  = Neurofeedback_PhysiologicalNoise(FreqSD, FreqMean, ResolutionStep, timestamps)
%% Version V1
% Authors - Mario De Los Santos, Felipe Orihuela-Espina, Javier
% Herrera-Vega, Javier Andreu-Pérez
% Date - July 18th, 2022
% Email - madlsh3517@gmail.com
% Based on: Elwell et. al., 1999. Oscillations in cerebal haemodynamics.
%
%% Input Parameters
% FreqSD - Frequency standard deviation of the physiological noise. Scalar
% FreqMean - Frequency Mean of the physiological noise. Scalar
% Resolution Step - Sampling rate. Scalar
% Timestamps - Time sequence for the stimulus train. <1 x simulationLength>
% NRegions - Number of regions activated. Scalar.
%% Output Parameters
% 
% HemoNoises -  Noise generation for the hemodynamics signals.
%               <NRegions x simulationLength>
%
%% 

%Variables to ADD the noises to the models. 
% These variables divide the hemodynamics 
% inputs depending on the number of regions.
HemoNoises = 0;
%
%Calculation of the operative ranges to use
Initial =  FreqMean - 2*FreqSD;
Ending = FreqMean +  2*FreqSD;
Calsize = (Ending - Initial - ResolutionStep)/ResolutionStep;
%Calsize = ResolutionStep;
FrequencySet = linspace(Initial, Ending, Calsize);

amplitudeScaling = 1;
theta = 0;
for i = 1:Calsize
    s = rng; %Rebot random seeed 
    %Random Amplitude
    %Centralized gaussian in the dispersion mean 
    %A = 0;
    A = amplitudeScaling * normrnd(FreqMean,FreqSD);
    %A = amplitudeScaling * rand(1);
    %Random phase
    %theta = 2 * pi * normrnd(FreqMean, FreqSD) - pi;
    
    %Fundamental signal
    tmpSin = A * sin(2*pi*(FrequencySet(1,i) * timestamps + theta));
    HemoNoises = HemoNoises + tmpSin;
end
%This section should be generalized but do the work for now.

== matlab function Neurofeedback_Fuzzy_MISO_Full_cute/Connectivity Extraction/getConnectivity ==
  data: D input; Bobs output; DQ output; Threshold input
function [Bobs,DQ]  = getConnectivity(D, Threshold)

    DQ = zeros(1, 2);
    DQ(1,1)=D(1,1);
    DQ(1,2)=D(1,2);


    DH = zeros(1,2);
    DH(1,1)=D(1,3);
    DH(1,2)=D(1,4);

    rThresh= Threshold; % [0..1] A threshold on the correlation.

    [~,nChannels, nHb]=size(DQ);

    C = nan(nChannels, nChannels, nHb); %Matrix of channel pairwise correlations;

    %This part of the algorithm is HIGHLY inefficient but it does the job for now
    %but might not be sufficiently fast for "real time" neurofeedback

    for iHb = 1:nHb
        for iCh=1:nChannels
            for jCh=iCh:nChannels

                if iCh == jCh

                 C(iCh,jCh,iHb) = 1;

                else

                 C(iCh,jCh,iHb) = xcorr2(DQ(:,iCh,iHb),DQ(:,jCh,iHb));

                end
            end

        end

    end

    %Threshold/Binarize C


    tmp = C > rThresh;

    %Finally "merge" accross Hb species

    Bobs = all(tmp,3); %Apply the AND function across Hb species.

== matlab function Neurofeedback_Fuzzy_MISO_Full_cute/fNIRS Processing/Channel Organizer ==
  data: u input; y output
function y = fcn(u)

y = [1; 2; 3; 4;];

y(1) = u(1,1);
y(2) = u(2,1);
y(3) = u(1,2);
y(4) = u(2,2);

== matlab function Neurofeedback_Fuzzy_MISO_Full_cute/Connectivity_Regions2 ==
  data: Bobs input; B_00 output; B_01 output; B_10 output; B_11 output
function [B_00, B_01, B_10, B_11] = fcn(Bobs)


B_00 = (Bobs(1,1));
B_01 = (Bobs(1,2));
B_10 = (Bobs(2,1));
B_11 = (Bobs(2,2));

== matlab function Neurofeedback_Fuzzy_MISO_Full_cute/Error Function2/Error Function/ErrorFunction_GRG ==
  data: Bref input; E output size=1; Bobs input; Pref input; Pobs input; SHD input; w1_l input; errP output; errA output
function [E, errP, errA]  = ErrorFunction(Bref, Bobs, Pref, Pobs, SHD, w1_l)
    w1 = w1_l; %Use whatever values you like most. Threshold 

    w2 = 1 - w1;

    assert(all(size(Bref) == size(Bobs)));

    assert(size(Bref,1) == size(Bref,2));

    nChannels = size(Bref,1);

    BfullyConnected = ones(nChannels);

    BfullyDisconnected = zeros(nChannels);

   
    maxDiffSHD= sum(sum(xor(BfullyConnected,BfullyDisconnected))); %SHD
    errA = SHD/maxDiffSHD; %Normalize error in the connectivity
    %errP = (abs(Pref-Pobs))/abs(Pref);
    %tmp = Pref;
    errP = abs(Pref-Pobs)/max(abs(Pref),1);

    
E = (w1 * errA + w2 * errP);

== matlab function Neurofeedback_Fuzzy_MISO_Full_cute/Connectivity Extraction/Incremental_Avg_Boot1/Reboot/MATLAB Function1 ==
  data: Timer input; Reset output; Cycle_time input; periods input
function Reset  = fcn(Timer, Cycle_time, periods)

temp = 0;
PCycles = zeros(periods,1);
for i = 1:periods
    PCycles(i) = i * Cycle_time;
    if (Timer >= PCycles(i) && Timer <= PCycles(i)+1)
        temp = 1;
        break
    else
        temp = 0;
    end
end 
Reset = temp;

== matlab function Neurofeedback_Fuzzy_MISO_Full_cute/Connectivity Extraction/Incremental_Avg_Boot1/Reboot/MATLAB Function2 ==
  data: reset input; y_s input; y output
function y = fcn(reset, y_s)

if reset == 1
    y = 0;
else 
    y = (y_s + 1);
end

== matlab function Neurofeedback_Fuzzy_MISO_Full_cute/Synthetic Human Agent/Hemodynamics/Rate Blood Volume/Fv_s ==
  data: Vj input; Vj_expphi output
function Vj_expphi = fcn(Vj)
phi = 0.32;
Vj_expphi = Vj.^(1/phi);

== matlab function Neurofeedback_Fuzzy_MISO_Full_cute/Synthetic Human Agent/Hemodynamics/Rate Blood Volume/Vj//Tjv ==
  data: Vj input; Vj_Tjv output
function Vj_Tjv = fcn(Vj)
    Tjv = 2*exp([0;1]);
    Tj = 2*exp([0;0.05]);
Vj_Tjv =(Tj.*Tjv.*Vj);

== matlab function Neurofeedback_Fuzzy_MISO_Full_cute/Synthetic Human Agent/Human_Pressure/Pressure Generator ==
  data: Zt input; Pobs output; t input
function Pobs = fcn(Zt, t)
    R=10000; %Resistor [Ohms];
    C= 2; %Capacitor [Faradays];
    V= Zt(1); %Voltage or system reference;
    Vc = V * (exp(-t/(R*C))); % Voltage at the capacitor  
    
Pobs = Vc;

== matlab function Neurofeedback_Fuzzy_MISO_Full_cute/Synthetic Human Agent/Human_Pressure/SENSOR ==
  data: Vout input; Pobs output
function Pobs  = PressureGenerator_sensor(Vout)

    Vcc = 50; %Considering 5V as a real sensor, the value is on mV
    Rf = 100; %Fixed resistor 10k ohms
    kgf = 0.1019716213; % 1N = 0.1019716213 kgf
    Fsr = 0;
    Fsrforce = 0;
    Fsr = (Vcc - Vout * Rf) / Vout;
    FsConductance = 1000000; %Sensor conductance in uOhms
    FsConductance = FsConductance / Fsr;
    if FsConductance <= 1000
        Fsrforce = FsConductance / 80; %Force on Newtons
    else
        Fsrforce = FsConductance - 1000;
        Fsrforce = Fsrforce / 30;
    end
    
Pobs = Fsrforce * kgf;

end

== matlab function Neurofeedback_Fuzzy_MISO_Full_cute/Synthetic Human Agent/Neurodynamics_Static/Jt ==
  data: Zt input; U input; Jt output; B_input input; A_input input
function Jt = fcn(Zt, U, B_input, A_input)
   A = A_input;
   nRegions  = size(A,1);
   M = size(U,1); %nStimuli
   simulationLength = size(U,2);
   %NOTE: Consider that in case of have more than one stimulus, you must
   %change this. 
   B = B_input;
   T = zeros(nRegions); %nRegions x nRegions
    for t = 1:simulationLength
           for uu = 1:M % Sum (Uj * Bj)
               tmp = U(uu,t)*B(:,:,uu);
               T = -0.5*exp(T + tmp);  
           end
    end
    SI = diag(A);
    A =  A - diag(exp(SI) + SI);
Jt = (A*Zt) + (T*Zt);

== matlab function Neurofeedback_Fuzzy_MISO_Full_cute/Synthetic Human Agent/Optics_ ==
  data: DH input; DQ input; Y output
function Y    = Optical_Changes(DH, DQ)
%% Version V1
% Authors - Mario De Los Santos, Felipe Orihuela-Espina, Javier Herrara-Vega
% Date - March, 2022
% Email - madlsh3517@gmail.com
% Based on: 2015 Stak DCM for fNIRS.
%
%% Input Parameters
% DQ - HbR - Rate of deoxy-hemoglobin
% DH - HbT - Total Hemoglobin
%
%% Output Parameters
% y- optical density changes 
%
%% 

%Using simulink is not possible to have a dynamic matrix that we can
%iterate based on the nRegions variable, but you could easly replace the
%number of regions in the variable "Regions" according your needs
Regions = 2;
Y = zeros(Regions,Regions);
Ytemp1 = zeros(Regions,1);
Ytemp2 = zeros(Regions,1);
tempDHQ = zeros(Regions, 2);

%Debug temporal
L1 = zeros(Regions, 1);
L2 = zeros(Regions, 1);

% We are using as L1 = 780nm and as L2 = 850nm (same as STak for the
% second one)
%Based on: Giannoni, L., Lange, F., & Tachtsidis, I. (2020). Investigation of the quantification 
% of hemoglobin and cytochrome-c-oxidase in the exposed cortex with near-infrared hyperspectral imaging: 
% a simulation study. Journal of biomedical optics, 25(4), 046001.


F_P =[(0.0007358251*7.5) (0.001104715*6.5);
      (0.001159306*7.5) (0.0007858993*6.5)];
%F_P = [(735.8251*7.5), (1104.715*7.5); (1159.306*7.5), (785.8993*7.5)];
%Itereation between regions, nRegions is given as constant by the user.

    tempDHQ(1,1) = DH(1);
    tempDHQ(1,2) = DH(2);

    tempDHQ(2,1) = DQ(1);
    tempDHQ(2,2) = DQ(2);


    Ytemp1 = F_P * tempDHQ(:,1);
    Ytemp2 = F_P * tempDHQ(:,2);

    Y(:,1) = Ytemp1;
    Y(:,2) = Ytemp2;

% L1(1,1) = Y(1,1);
% L1(2,1) = Y(1,2);
% 
% L2(1,1) = Y(2,1);
% L2(2,1) = Y(2,2);

== matlab function Neurofeedback_Fuzzy_MISO_Full_cute/fNIRS Processing/MATLAB Function2 ==
  data: e_coefficients input; A output; DPF input
function A  = A(e_coefficients, DPF)
%Molar extinction coefficients 
%Considering the wavelengths of the STak implentation, we need to use
% 780nm and 850nm

%780nm = [735.8251 1104.715];
%850nm = [1159.306 785.8993];
%e_coefficients = [735.8251 1104.715;
 %                   1159.306 785.8993];

% https://mail.nmr.mgh.harvard.edu/pipermail//homer-users/2006-July/000124.html
%Differential Path Lenght
%NOTE: need to confirm this, I'm taking the values from an old
%implementation
%DPF = [10.3; 8.4];

%Distance; this is an assumption of 3cm
%Distance = 3;
A = [e_coefficients(1, 1)*DPF(1), e_coefficients(1, 2)*DPF(1);...
    e_coefficients(2, 1)*DPF(2), e_coefficients(2, 1)*DPF(2)];

== matlab function Neurofeedback_Fuzzy_MISO_Full_cute/Error Function2/Error Function/MATLAB Function(err2)_Saturated ==
  data: Bref input; E output size=1; Bobs input; Pref input; Pobs input; SHD input; w1_l input; errP output; errA output
function [E, errP, errA]  = ErrorFunction(Bref, Bobs, Pref, Pobs, SHD, w1_l)
    w1 = w1_l; %Use whatever values you like most. Threshold 

    w2 = 1 - w1;

    assert(all(size(Bref) == size(Bobs)));

    assert(size(Bref,1) == size(Bref,2));

    nChannels = size(Bref,1);

    BfullyConnected = ones(nChannels);

    BfullyDisconnected = zeros(nChannels);

   
    maxDiffSHD= sum(sum(xor(BfullyConnected,BfullyDisconnected))); %SHD
    errA = SHD/maxDiffSHD; %Normalize error in the connectivity
    %errP = (abs(Pref-Pobs))/abs(Pref);
    %tmp = Pref;
    errP = 0;
    if Pref == 0
        Pref = 0.0005;
    else
        %errP = abs(Pref-Pobs)/abs(Pref);
        errP = exp (1 / abs(Pref-Pobs)/abs(Pref));
      if errP > 1
            errP = 1;
      end
    end
    %errP = (abs(Pref-Pobs))/abs(tmp);
    
    
E = (w1 * errA + w2 * errP);

== matlab function Neurofeedback_Fuzzy_MISO_Full_cute/Synthetic Human Agent/Neurodynamics_Static/B_Dynamic/MATLAB Function ==
  settings: updateMethod=DISCRETE
  data: B input; B_d output; U input; Th output; T input; B_D input; Th_O input
function [B_d, Th]= fcn(B, U, T,B_D, Th_O)
B_d = zeros(2,2);
Th = [1 1 1 1; 1 1 1 1];
down = -1;
up = 1;
%Plasticity threshold
if T >= 0 && T <= 1
    x = rand(1, 4);
    x = sort(x);
    s = std(x);
    Th(1,:) = x;
    Th(2,:) = x + s;
else
    Th = Th_O;
end
db = B;
if U > Th(1,2) && U < Th(2, 2)
   dB = (up-down).*rand(2,2) + down;
   if(det(dB) > 0.3 && det(db) < 0.5)
       B_d = dB;
   else
       dB = (up-down).*rand(2,2) + down;
       B_d = dB;
   end
elseif U > Th(2,2) && U < Th(1,3)
   dB = (up-down).*rand(2,2) + down;
   if(det(dB) > 0 && det(db) < 0.3)
       B_d = dB;
   else
       dB = (up-down).*rand(2,2) + down;
       B_d = dB;
   end
else
    B_d = B;
end

== matlab function Neurofeedback_Fuzzy_MISO_Full_cute/Synthetic Human Agent/DH and DQ/MATLAB Function1 ==
  data: DH1 input; H output; DH2 input; DQ1 input; DQ2 input
function H = hemo(DH1, DH2, DQ1, DQ2)
H = zeros(1,4);

H(1,1) = DQ1;
H(1,2) = DQ2;
H(1,3) = DH1;
H(1,4) = DH2;

== matlab function Neurofeedback_Fuzzy_MISO_Full_cute/Error Function2/Error Function/Error_SHD ==
  data: Aref input; val output; Aobs input; matrix output
function [val,matrix]=SHD(Aref,Aobs)

val = sum(sum(xor(Aref,Aobs)));
matrix = xor(Aref,Aobs);

== matlab function Neurofeedback_Fuzzy_MISO_Full_cute/Synthetic Human Agent/Hemodynamics/Efp ==
  data: fjin input; Efp output
function Efp= fcn(fjin)

Efp = (1 - (1 - 0.32).^ (1 ./ fjin))/0.32;

== matlab function Neurofeedback_Fuzzy_MISO_Full_cute/fNIRS Processing/Modified Beer Lamber Law ==
  data: OD input; Hemodynamics output; A input
function Hemodynamics = MBLL(OD, A)

% B = zeros(2,2);
% 
% B(1, 1) = Delta1(1, 1);
% B(1, 2) = Delta1(2, 1);
% 
% B(2, 1) = Delta2(1, 1);
% B(2, 2) = Delta2(2, 1);

Hemodynamics = (A\OD)';
